simulink subsystem "InversePendulum2022"  (R2022b)
settings: Solver=VariableStepAuto  StartTime=0.0  StopTime=10.0  RelTol=1e-3
undefined symbols (not defined in the file): A, B, g, I, Init_St, l, m, M, p
settings Model: Creator=Лиза  LastModifiedBy=romav
settings OptimizationCC: ReuseModelBlockBuffer=on

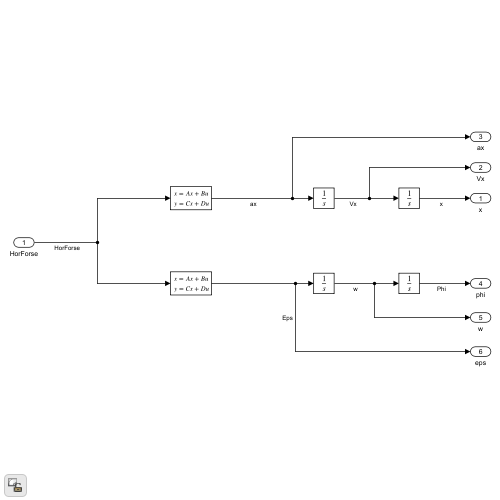
[thumbnail: Simulink's stored preview of the top-level diagram]
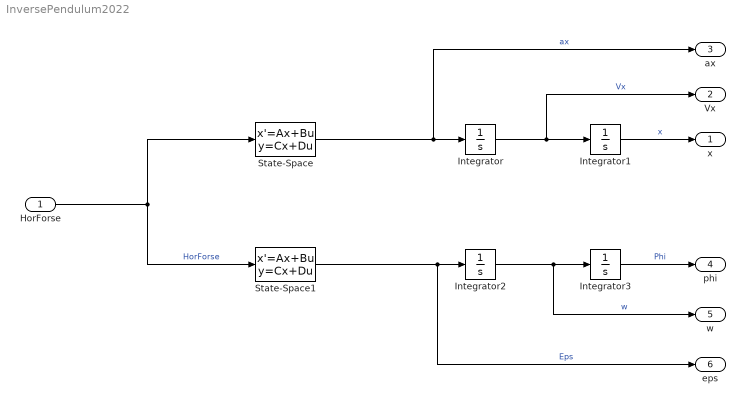
== system InversePendulum2022 ==
  HorForse : Inport
  Integrator{,1..3} (4 alike) : Integrator
  State-Space : StateSpace  A=A  B=B  C="[ 0      0          (m^2*g*l^2)/p   0]"  D=[(I+m*l^2)/p]  InitialCondition=Init_St
  State-Space1 : StateSpace  A=A  B=B  C=[ 0 0 -m*g*l*(M+m)/p 0]  D=-m*l/p  InitialCondition=Init_St
  x : Outport
  Vx : Outport  Port=2
  ax : Outport  Port=3
  phi : Outport  Port=4
  w : Outport  Port=5
  eps : Outport  Port=6
  wires:
  HorForse/1 -> State-Space1/1, State-Space/1  "HorForse"
  State-Space/1 -> ax/1, Integrator/1  "ax"
  Integrator/1 -> Vx/1, Integrator1/1  "Vx"
  State-Space1/1 -> eps/1, Integrator2/1  "Eps"
  Integrator2/1 -> w/1, Integrator3/1  "w"
  Integrator1/1 -> x/1  "x"
  Integrator3/1 -> phi/1  "Phi"
